simulink model "ICE_and_EM_Power"  (R2013a)
settings: Solver=ode45  StartTime=0.0  StopTime=10.0  RelTol=1e-3
libraries: simulink x1
settings Model: Creator=Admin  LastModifiedBy=Admin

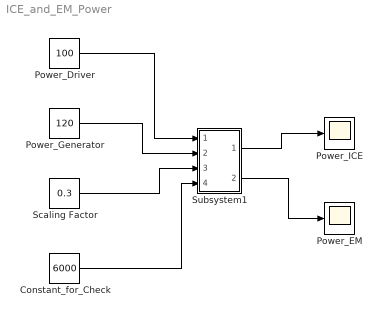
== system ICE_and_EM_Power ==
  Constant_for_Check : Constant  Value=6000
  Power_Driver : Constant  Value=100
  Power_EM : Scope
  Power_Generator : Constant  Value=120
  Power_ICE : Scope
  Scaling Factor : Constant  Value=0.3
  Subsystem1 : Subsystem
  wires:
  Power_Driver/1 -> Subsystem1/1(In1)
  Power_Generator/1 -> Subsystem1/2(In2)
  Scaling Factor/1 -> Subsystem1/3(In3)
  Constant_for_Check/1 -> Subsystem1/4(In4)
  Subsystem1/1(Out1) -> Power_ICE/1
  Subsystem1/2(Out2) -> Power_EM/1

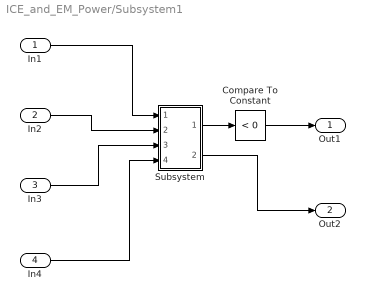
== system ICE_and_EM_Power/Subsystem1 ==
  In1 : Inport
  In2 : Inport  Port=2
  In3 : Inport  Port=3
  In4 : Inport  Port=4
  Compare To Constant : simulink/Logic and Bit Operations/Compare To Constant  relop=<  const=0  OutDataTypeStr=boolean
  Subsystem : Subsystem
  Out1 : Outport
  Out2 : Outport  Port=2
  wires:
  Subsystem/2(Out2) -> Out2/1
  In4/1 -> Subsystem/4(In4)
  Compare To Constant/1 -> Out1/1
  In3/1 -> Subsystem/3(In3)
  In1/1 -> Subsystem/1(In1)
  In2/1 -> Subsystem/2(In2)
  Subsystem/1(Out1) -> Compare To Constant/1

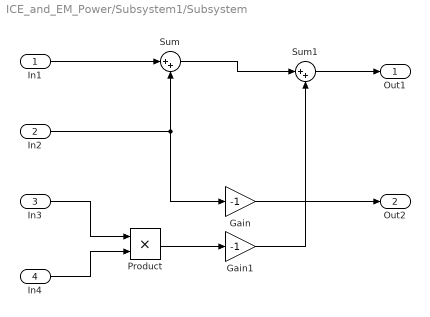
== system ICE_and_EM_Power/Subsystem1/Subsystem ==
  In1 : Inport
  In2 : Inport  Port=2
  In3 : Inport  Port=3
  In4 : Inport  Port=4
  Gain : Gain  Gain=-1
  Gain1 : Gain  Gain=-1
  Product : Product
  Sum : Sum  Inputs=|++
  Sum1 : Sum  Inputs=|++
  Out1 : Outport
  Out2 : Outport  Port=2
  wires:
  Product/1 -> Gain1/1
  In3/1 -> Product/1
  Sum/1 -> Sum1/1
  In4/1 -> Product/2
  Sum1/1 -> Out1/1
  In2/1 -> Gain/1, Sum/2
  Gain1/1 -> Sum1/2
  Gain/1 -> Out2/1
  In1/1 -> Sum/1
